simulink model "tutorial15_codegen"  (R2025a)
settings: Solver=VariableStepAuto  StartTime=0.0  StopTime=10.0  RelTol=1e-3
settings Model: Creator=xing2  LastModifiedBy=xing2

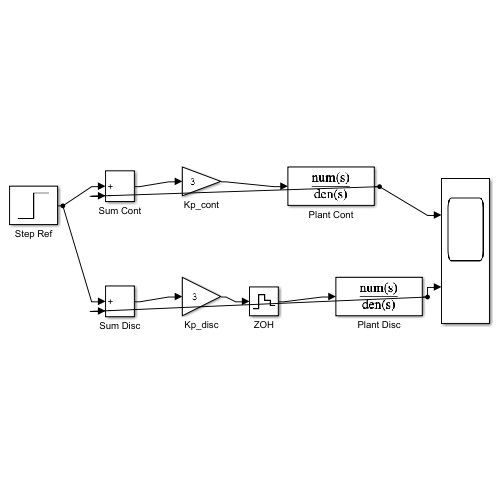
[thumbnail: Simulink's stored preview of the top-level diagram]
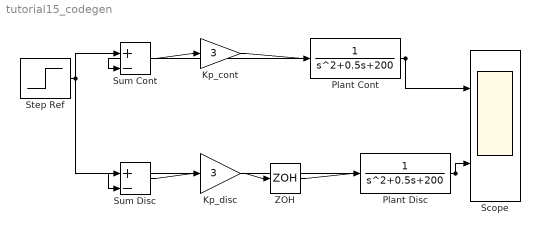
== system tutorial15_codegen ==
  Kp_cont : Gain  Gain=3
  Kp_disc : Gain  Gain=3
  Plant Cont : TransferFcn  Denominator=[1 0.5 200]
  Plant Disc : TransferFcn  Denominator=[1 0.5 200]
  Scope : Scope  NumInputPorts=2
  Step Ref : Step  Time=0.5  SampleTime=0
  Sum Cont : Sum  Inputs=|+-
  Sum Disc : Sum  Inputs=|+-
  ZOH : ZeroOrderHold  SampleTime=0.005
  wires:
  Step Ref/1 -> Sum Cont/1, Sum Disc/1
  Sum Cont/1 -> Kp_cont/1
  Kp_cont/1 -> Plant Cont/1
  Plant Cont/1 -> Scope/1, Sum Cont/2
  Sum Disc/1 -> Kp_disc/1
  Kp_disc/1 -> ZOH/1
  ZOH/1 -> Plant Disc/1
  Plant Disc/1 -> Scope/2, Sum Disc/2
